simulink model "a8_AnregungReibung_lsgFcnBlock"  (R2020b)
settings: Solver=ode45  StartTime=0.0  StopTime=50.0  MaxStep=0.1  RelTol=1e-3
model workspace (MAT data in the model file):
  d = 0.4
  w = 1
  w0 = 2.2360679775
settings Model: Creator=Reichl  LastModifiedBy=jakob
settings DataIOCC: ReturnWorkspaceOutputs=off
settings DebuggingCC: ArithmeticOperatorsInVariantConditions=warning
settings SFSimCC: SimUseLocalCustomCode=off  CustomCodeUndefinedFunction=UseInterfaceOnly
settings RTWCC: RTWUseLocalCustomCode=off
settings CodeAppCC: StateflowObjectComments=on

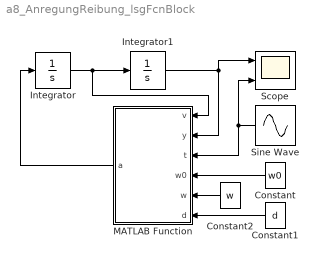
== system a8_AnregungReibung_lsgFcnBlock ==
  Constant : Constant  Value=w0
  Constant1 : Constant  Value=d
  Constant2 : Constant  Value=w
  Integrator : Integrator
  Integrator1 : Integrator
  MATLAB Function : MATLAB Function  TreatAsAtomicUnit=on
  Scope : Scope  NumInputPorts=2
  Sine Wave : Sin  Frequency=w  SampleTime=0
  wires:
  Integrator/1 -> Integrator1/1, MATLAB Function/1(v)
  Integrator1/1 -> Scope/1, MATLAB Function/2(y)
  Sine Wave/1 -> Scope/2, MATLAB Function/3(t)
  Constant/1 -> MATLAB Function/4(w0)
  Constant1/1 -> MATLAB Function/6(d)
  Constant2/1 -> MATLAB Function/5(w)
  MATLAB Function/1(a) -> Integrator/1

== matlab function a8_AnregungReibung_lsgFcnBlock/MATLAB Function ==
  data: v input; a output; y input; t input; w0 input; w input; d input
function a = fcn(v,y,t,w0,w,d)

if v>0
   vz = 1.0;
elseif v <0
   vz = -1.0;
else
   vz = 0.0;
end
a = -vz*d*v*v-w0*w0*y+sin(w*t);
